simulink model "f_22_stabilator_control - Copy"  (R2025b)
settings: Solver=ode23t  StartTime=0.0  StopTime=10.0  MinStep=1e-8  RelTol=1e-3  AbsTol=1e-6
InitFcn:
  | Running_in_Simulink = 1;
  | 
  | Relation;
values from neighbouring files (symbols this model uses):
  alpha = rad2deg(asin(d/a))    [Relation.m]
  D = 163.1    [EHA_initialization.m]
  deflection = deflection_min:0.01:deflection_max    [Relation.m]
  extension = sqrt(a^2 + r^2 - 2.*a.*r.*cos(deg2rad(alpha-deflection))) - d    [Relation.m]
  F_act = M_pivot ./ lever_arm_actuator    [Relation.m]
  J = 0.205    [EHA_initialization.m]
  K_e = 0.132    [EHA_initialization.m]
  K_vism = 1    [EHA_initialization.m]
  L = 1.95e-5    (= 1.95e-05)    [EHA_initialization.m]
  P_aci = P_acnom    (= 20.7)    [EHA_initialization.m]
  R = 138000/(370^2)    (= 1.00803506209)    [EHA_initialization.m]
  V_gasi = V_gasnom    (= 0.00206)    [EHA_initialization.m]
  velocity = 300    [Relation.m]
undefined symbols (not defined in the file or in its folder): A, B, beta, F_c, F_s, k, K_elp, K_ilj, K_ilp, K_t, K_vis, M, T_c, T_f, V_10, V_20
libraries: slpidlib x3
settings Model: Creator=Arseni  LastModifiedBy=User
settings SolverCC: AutoScaleAbsTol=off  MaxConsecutiveMinStep=10  SolverResetMethod=Robust

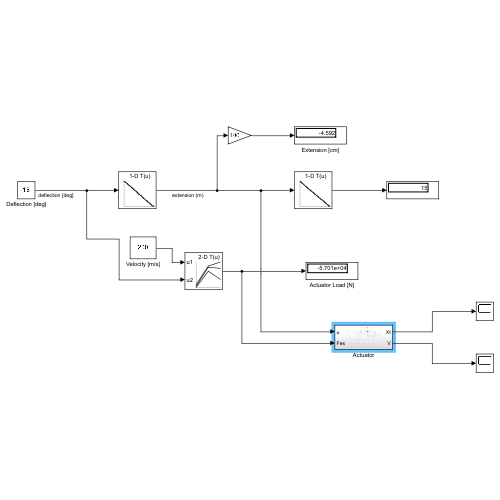
[thumbnail: Simulink's stored preview of the top-level diagram]
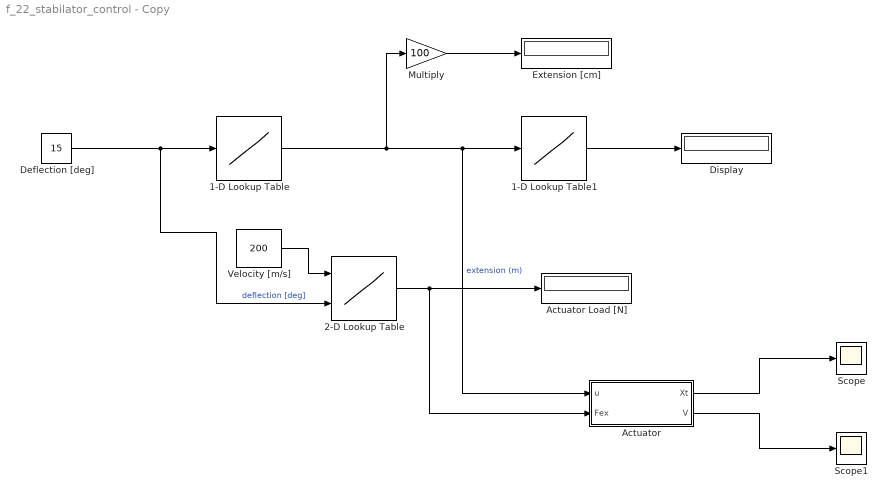
== system f_22_stabilator_control - Copy ==
  1-D Lookup Table : Lookup_n-D  NumberOfTableDimensions=1  BreakpointsForDimension1=deflection  Table=extension  InternalRulePriority=Speed  RndMeth=Simplest
  1-D Lookup Table1 : Lookup_n-D  NumberOfTableDimensions=1  BreakpointsForDimension1=flip(extension)  Table=flip(deflection)  InternalRulePriority=Speed  RndMeth=Simplest
  2-D Lookup Table : Lookup_n-D  BreakpointsForDimension1=velocity  BreakpointsForDimension2=deflection  Table=F_act  InternalRulePriority=Speed  RndMeth=Simplest
      settings: InputPortMap=u0,u1
  Actuator : Subsystem
  Actuator Load [N] : Display
  Deflection [deg] : Constant  Value=15
  Display : Display
  Extension [cm] : Display
  Multiply : Gain  Gain=100
  Scope : Scope
      settings: ActiveDisplayYMinimum=-0.010270198712265704  ActiveDisplayYMaximum=0.016528927509019922
  Scope1 : Scope
      settings: ActiveDisplayYMinimum=-22.309265699882108  ActiveDisplayYMaximum=23.598774285341456
  Velocity [m/s] : Constant  Value=200
  wires:
  Deflection [deg]/1 -> 2-D Lookup Table/2, 1-D Lookup Table/1  "deflection [deg]"
  1-D Lookup Table/1 -> 1-D Lookup Table1/1, Actuator/1(u), Multiply/1  "extension (m)"
  1-D Lookup Table1/1 -> Display/1
  Multiply/1 -> Extension [cm]/1
  2-D Lookup Table/1 -> Actuator Load [N]/1, Actuator/2(Fex)
  Velocity [m/s]/1 -> 2-D Lookup Table/1
  Actuator/1(Xt) -> Scope/1
  Actuator/2(V) -> Scope1/1

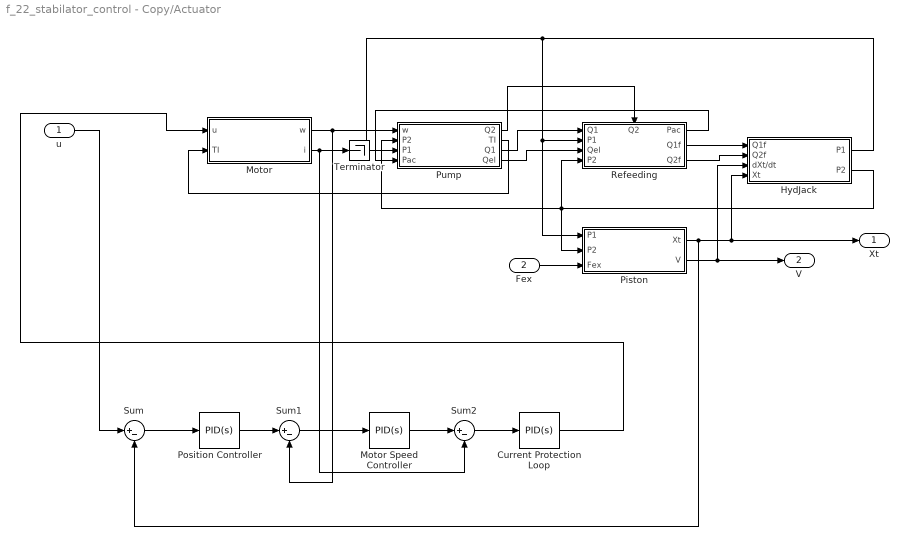
== system f_22_stabilator_control - Copy/Actuator ==
  u : Inport
  Fex : Inport  Port=2
  Current Protection Loop : slpidlib/PID Controller  Controller=PID  Form=Parallel  TimeDomain=Continuous-time  UseExternalTs=off  SampleTime=-1  IntegratorMethod=Forward Euler  FilterMethod=Forward Euler  ControllerParametersSource=internal  P=0.5  I=0  UseKiTs=off  D=0  UseExternalDerivativeSource=off  N=100  UseFilter=on  TunerSelectOption=Transfer Function Based (PID Tuner App)  InitialConditionSource=internal  InitialConditionForIntegrator=0  InitialConditionForFilter=0  DifferentiatorICPrevScaledInput=0  ExternalReset=none  TrackingMode=off  Kt=1  LimitOutput=on  SatLimitsSource=internal  UpperSaturationLimit=270  LowerSaturationLimit=-270  LinearizeAsGain=on  AntiWindupMode=clamping  Kb=1  LimitIntegrator=off  UpperIntegratorSaturationLimit=inf  LowerIntegratorSaturationLimit=-inf  POutMin=[]  POutMax=[]  IOutMin=[]  IOutMax=[]  DOutMin=[]  DOutMax=[]  NOutMin=[]  NOutMax=[]  SumOutMin=[]  SumOutMax=[]  SaturationOutMin=[]  SaturationOutMax=[]  PParamMin=[]  PParamMax=[]  IParamMin=[]  IParamMax=[]  DParamMin=[]  DParamMax=[]  NParamMin=[]  NParamMax=[]  KbParamMin=[]  KbParamMax=[]  KtParamMin=[]  KtParamMax=[]  KbOutMin=[]  KbOutMax=[]  KtOutMin=[]  KtOutMax=[]  IntegratorOutMin=[]  IntegratorOutMax=[]  FilterOutMin=[]  FilterOutMax=[]  SumI1OutMin=[]  SumI1OutMax=[]  SumI2OutMin=[]  SumI2OutMax=[]  SumI3OutMin=[]  SumI3OutMax=[]  SumI4OutMin=[]  SumI4OutMax=[]  SumDOutMin=[]  SumDOutMax=[]  DifferentiatorOutMin=[]  DifferentiatorOutMax=[]  FilterDiffOutCoefMin=[]  FilterDiffOutCoefMax=[]  ReciprocalOutMin=[]  ReciprocalOutMax=[]  SumDenOutMin=[]  SumDenOutMax=[]  SumNumOutMin=[]  SumNumOutMax=[]  DivideOutMin=[]  DivideOutMax=[]  UdiffTsProdOutMin=[]  UdiffTsProdOutMax=[]  NTsProdOutMin=[]  NTsProdOutMax=[]  UintegralTsProdOutMin=[]  UintegralTsProdOutMax=[]  UngainTsProdOutMin=[]  UngainTsProdOutMax=[]  ClampingZeroOutDataTypeStr=Inherit: Inherit via back propagation  ClampingZeroOutMin=[]  ClampingZeroOutMax=[]  FilterDenConstantOutDataTypeStr=Inherit: Inherit via back propagation  FilterDenConstantOutMin=[]  FilterDenConstantOutMax=[]  PCopyOutDataTypeStr=Inherit: Inherit via back propagation  PCopyOutMin=[]  PCopyOutMax=[]  NCopyOutDataTypeStr=Inherit: Inherit via back propagation  NCopyOutMin=[]  NCopyOutMax=[]  IntegratorContinuousStateAttributes=''  IntegratorStateMustResolveToSignalObject=off  IntegratorRTWStateStorageClass=Auto  FilterContinuousStateAttributes=''  FilterStateMustResolveToSignalObject=off  FilterRTWStateStorageClass=Auto  ParallelPVariant=InternalParameters  IdealPVariant=Disabled  IVariant=InternalParameters  DVariant=InternalParameters  IntegratorVariant=Continuous  SatVariant=Enabled  AWVariant=ContClampingParallel  PCopyVariant=Disabled  TRVariant=Disabled  FdbkBlocksVariant=Forward  IdealPFdbkVariant=Disabled  SatFdbkVariant=Disabled  DerivativeFilterVariant=ContFilter  NVariant=InternalParameters  NCopyVariant=Disabled  FilterICVariant=InternalICsFilter  IntegratorICVariant=InternalICs  ExternalResetVariant=Disabled  TRSumVariant=Passthrough  SumFdbkVariant=Disabled  SumVariant=Sum_PID  TsampFilterVariant=InternalTs  TsampNgainVariant=Passthrough  TsampIntegralVariant=Disabled_SignalSpec  ExternalSaturationOutDataTypeStr=Inherit: Same as second input  DerivativeSourceVariant=ErrorSignal  PreIntVariant=InternalPreInt
  HydJack : Subsystem
  Motor : Subsystem
  Motor Speed Controller : slpidlib/PID Controller  Controller=PID  Form=Parallel  TimeDomain=Continuous-time  UseExternalTs=off  SampleTime=-1  IntegratorMethod=Forward Euler  FilterMethod=Forward Euler  ControllerParametersSource=internal  P=5  I=1  UseKiTs=off  D=1  UseExternalDerivativeSource=off  N=100  UseFilter=on  TunerSelectOption=Transfer Function Based (PID Tuner App)  InitialConditionSource=internal  InitialConditionForIntegrator=0  InitialConditionForFilter=0  DifferentiatorICPrevScaledInput=0  ExternalReset=none  TrackingMode=off  Kt=1  LimitOutput=off  SatLimitsSource=internal  UpperSaturationLimit=inf  LowerSaturationLimit=-inf  LinearizeAsGain=on  AntiWindupMode=none  Kb=1  LimitIntegrator=off  UpperIntegratorSaturationLimit=inf  LowerIntegratorSaturationLimit=-inf  POutMin=[]  POutMax=[]  IOutMin=[]  IOutMax=[]  DOutMin=[]  DOutMax=[]  NOutMin=[]  NOutMax=[]  SumOutMin=[]  SumOutMax=[]  SaturationOutMin=[]  SaturationOutMax=[]  PParamMin=[]  PParamMax=[]  IParamMin=[]  IParamMax=[]  DParamMin=[]  DParamMax=[]  NParamMin=[]  NParamMax=[]  KbParamMin=[]  KbParamMax=[]  KtParamMin=[]  KtParamMax=[]  KbOutMin=[]  KbOutMax=[]  KtOutMin=[]  KtOutMax=[]  IntegratorOutMin=[]  IntegratorOutMax=[]  FilterOutMin=[]  FilterOutMax=[]  SumI1OutMin=[]  SumI1OutMax=[]  SumI2OutMin=[]  SumI2OutMax=[]  SumI3OutMin=[]  SumI3OutMax=[]  SumI4OutMin=[]  SumI4OutMax=[]  SumDOutMin=[]  SumDOutMax=[]  DifferentiatorOutMin=[]  DifferentiatorOutMax=[]  FilterDiffOutCoefMin=[]  FilterDiffOutCoefMax=[]  ReciprocalOutMin=[]  ReciprocalOutMax=[]  SumDenOutMin=[]  SumDenOutMax=[]  SumNumOutMin=[]  SumNumOutMax=[]  DivideOutMin=[]  DivideOutMax=[]  UdiffTsProdOutMin=[]  UdiffTsProdOutMax=[]  NTsProdOutMin=[]  NTsProdOutMax=[]  UintegralTsProdOutMin=[]  UintegralTsProdOutMax=[]  UngainTsProdOutMin=[]  UngainTsProdOutMax=[]  ClampingZeroOutDataTypeStr=Inherit: Inherit via back propagation  ClampingZeroOutMin=[]  ClampingZeroOutMax=[]  FilterDenConstantOutDataTypeStr=Inherit: Inherit via back propagation  FilterDenConstantOutMin=[]  FilterDenConstantOutMax=[]  PCopyOutDataTypeStr=Inherit: Inherit via back propagation  PCopyOutMin=[]  PCopyOutMax=[]  NCopyOutDataTypeStr=Inherit: Inherit via back propagation  NCopyOutMin=[]  NCopyOutMax=[]  IntegratorContinuousStateAttributes=''  IntegratorStateMustResolveToSignalObject=off  IntegratorRTWStateStorageClass=Auto  FilterContinuousStateAttributes=''  FilterStateMustResolveToSignalObject=off  FilterRTWStateStorageClass=Auto  ParallelPVariant=InternalParameters  IdealPVariant=Disabled  IVariant=InternalParameters  DVariant=InternalParameters  IntegratorVariant=Continuous  SatVariant=Disabled  AWVariant=Passthrough  PCopyVariant=Disabled  TRVariant=Disabled  FdbkBlocksVariant=Forward  IdealPFdbkVariant=Disabled  SatFdbkVariant=Disabled  DerivativeFilterVariant=ContFilter  NVariant=InternalParameters  NCopyVariant=Disabled  FilterICVariant=InternalICsFilter  IntegratorICVariant=InternalICs  ExternalResetVariant=Disabled  TRSumVariant=Passthrough  SumFdbkVariant=Disabled  SumVariant=Sum_PID  TsampFilterVariant=InternalTs  TsampNgainVariant=Passthrough  TsampIntegralVariant=Disabled_SignalSpec  ExternalSaturationOutDataTypeStr=Inherit: Same as second input  DerivativeSourceVariant=ErrorSignal  PreIntVariant=InternalPreInt
  Piston : Subsystem
  Position Controller : slpidlib/PID Controller  Controller=PID  Form=Parallel  TimeDomain=Continuous-time  UseExternalTs=off  SampleTime=-1  IntegratorMethod=Forward Euler  FilterMethod=Forward Euler  ControllerParametersSource=internal  P=0.5  I=0.1  UseKiTs=off  D=0  UseExternalDerivativeSource=off  N=100  UseFilter=on  TunerSelectOption=Transfer Function Based (PID Tuner App)  InitialConditionSource=internal  InitialConditionForIntegrator=0  InitialConditionForFilter=0  DifferentiatorICPrevScaledInput=0  ExternalReset=none  TrackingMode=off  Kt=1  LimitOutput=off  SatLimitsSource=internal  UpperSaturationLimit=inf  LowerSaturationLimit=-inf  LinearizeAsGain=on  AntiWindupMode=none  Kb=1  LimitIntegrator=off  UpperIntegratorSaturationLimit=inf  LowerIntegratorSaturationLimit=-inf  POutMin=[]  POutMax=[]  IOutMin=[]  IOutMax=[]  DOutMin=[]  DOutMax=[]  NOutMin=[]  NOutMax=[]  SumOutMin=[]  SumOutMax=[]  SaturationOutMin=[]  SaturationOutMax=[]  PParamMin=[]  PParamMax=[]  IParamMin=[]  IParamMax=[]  DParamMin=[]  DParamMax=[]  NParamMin=[]  NParamMax=[]  KbParamMin=[]  KbParamMax=[]  KtParamMin=[]  KtParamMax=[]  KbOutMin=[]  KbOutMax=[]  KtOutMin=[]  KtOutMax=[]  IntegratorOutMin=[]  IntegratorOutMax=[]  FilterOutMin=[]  FilterOutMax=[]  SumI1OutMin=[]  SumI1OutMax=[]  SumI2OutMin=[]  SumI2OutMax=[]  SumI3OutMin=[]  SumI3OutMax=[]  SumI4OutMin=[]  SumI4OutMax=[]  SumDOutMin=[]  SumDOutMax=[]  DifferentiatorOutMin=[]  DifferentiatorOutMax=[]  FilterDiffOutCoefMin=[]  FilterDiffOutCoefMax=[]  ReciprocalOutMin=[]  ReciprocalOutMax=[]  SumDenOutMin=[]  SumDenOutMax=[]  SumNumOutMin=[]  SumNumOutMax=[]  DivideOutMin=[]  DivideOutMax=[]  UdiffTsProdOutMin=[]  UdiffTsProdOutMax=[]  NTsProdOutMin=[]  NTsProdOutMax=[]  UintegralTsProdOutMin=[]  UintegralTsProdOutMax=[]  UngainTsProdOutMin=[]  UngainTsProdOutMax=[]  ClampingZeroOutDataTypeStr=Inherit: Inherit via back propagation  ClampingZeroOutMin=[]  ClampingZeroOutMax=[]  FilterDenConstantOutDataTypeStr=Inherit: Inherit via back propagation  FilterDenConstantOutMin=[]  FilterDenConstantOutMax=[]  PCopyOutDataTypeStr=Inherit: Inherit via back propagation  PCopyOutMin=[]  PCopyOutMax=[]  NCopyOutDataTypeStr=Inherit: Inherit via back propagation  NCopyOutMin=[]  NCopyOutMax=[]  IntegratorContinuousStateAttributes=''  IntegratorStateMustResolveToSignalObject=off  IntegratorRTWStateStorageClass=Auto  FilterContinuousStateAttributes=''  FilterStateMustResolveToSignalObject=off  FilterRTWStateStorageClass=Auto  ParallelPVariant=InternalParameters  IdealPVariant=Disabled  IVariant=InternalParameters  DVariant=InternalParameters  IntegratorVariant=Continuous  SatVariant=Disabled  AWVariant=Passthrough  PCopyVariant=Disabled  TRVariant=Disabled  FdbkBlocksVariant=Forward  IdealPFdbkVariant=Disabled  SatFdbkVariant=Disabled  DerivativeFilterVariant=ContFilter  NVariant=InternalParameters  NCopyVariant=Disabled  FilterICVariant=InternalICsFilter  IntegratorICVariant=InternalICs  ExternalResetVariant=Disabled  TRSumVariant=Passthrough  SumFdbkVariant=Disabled  SumVariant=Sum_PID  TsampFilterVariant=InternalTs  TsampNgainVariant=Passthrough  TsampIntegralVariant=Disabled_SignalSpec  ExternalSaturationOutDataTypeStr=Inherit: Same as second input  DerivativeSourceVariant=ErrorSignal  PreIntVariant=InternalPreInt
  Pump : Subsystem
  Refeeding : Subsystem
      settings: PortSchema="{\"entries\":[{\"content\":{\"sides\":[{\"content\":{\"connectorIds\":[\"In1\",\"In2\",\"In3\",\"In4\"]},\"type\":\"ConnectorPlacement.EquallySpacedRectSide\",\"uuid\":\"b1abc16c-430b-4270-8249-0157d5dcf7da\"},{\"content\":{\"connectorIds\":[\"Out1\",\"Out2\",\"Out3\"],\"side\":\"RIGHT\"},\"type\":\"ConnectorPlacement.EquallySpacedRectSide\",\"uuid\":\"915786c5-2ea2-4759-aadd-eadd86a3997f\"},{\"content\":{\"connectorIds\":[\"In5\"],\"side\":\"TOP\"},\"type\":\"ConnectorPlacement.EquallySpacedRectSide\",\"uuid\":\"af1c57d2-4a41-47dc-aec2-d26e5b158527\"}]},\"type\":\"ConnectorPlacement.EquallySpacedConnector\",\"uuid\":\"dcd4a5ce-5031-43e1-ac08-793124a08eaa\"}],\"packageUris\":[\"http://schema.mathworks.com/mf0/Connector/R2020b\"],\"version\":\"1.0\"}"
  Sum : Sum  Inputs=|+-
  Sum1 : Sum  Inputs=|+-
  Sum2 : Sum  Inputs=|+-
  Terminator : Terminator
  Xt : Outport
  V : Outport  Port=2
  wires:
  Motor/1(w) -> Pump/1(w), Sum1/2
  Motor/2(i) -> Terminator/1, Sum2/2
  Pump/3(Q1) -> Refeeding/1(Q1)
  Pump/1(Q2) -> Refeeding/5(Q2)
  Pump/4(Qel) -> Refeeding/3(Qel)
  Refeeding/1(Pac) -> Pump/4(Pac)
  Pump/2(TI) -> Motor/2(TI)
  Refeeding/2(Q1f) -> HydJack/1(Q1f)
  Refeeding/3(Q2f) -> HydJack/2(Q2f)
  HydJack/1(P1) -> Piston/1(P1), Refeeding/2(P1), Pump/3(P1)
  HydJack/2(P2) -> Refeeding/4(P2), Pump/2(P2), Piston/2(P2)
  Fex/1 -> Piston/3(Fex)
  Piston/1(Xt) -> Xt/1, HydJack/4(Xt), Sum/2
  Piston/2(V) -> V/1, HydJack/3(dXt/dt)
  u/1 -> Sum/1
  Sum/1 -> Position Controller/1
  Position Controller/1 -> Sum1/1
  Sum1/1 -> Motor Speed Controller/1
  Motor Speed Controller/1 -> Sum2/1
  Sum2/1 -> Current Protection Loop/1
  Current Protection Loop/1 -> Motor/1(u)

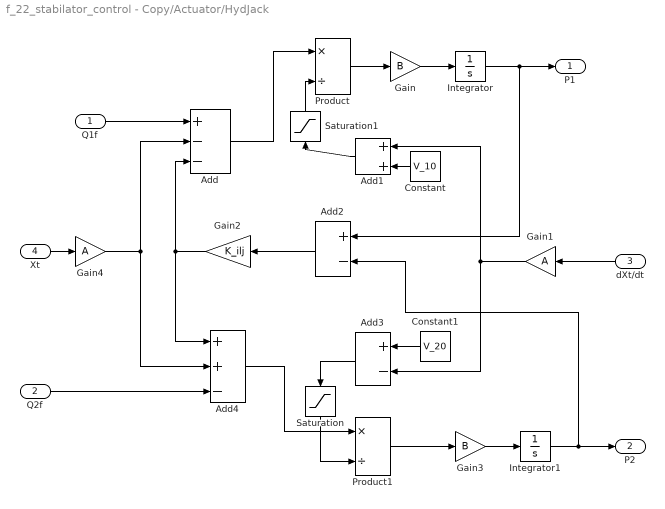
== system f_22_stabilator_control - Copy/Actuator/HydJack ==
  Q1f : Inport
  Q2f : Inport  Port=2
  dXt/dt : Inport  Port=3
  Xt : Inport  Port=4
  Add : Sum  Inputs=+--
  Add1 : Sum
  Add2 : Sum  Inputs=+-
  Add3 : Sum  Inputs=+-
  Add4 : Sum  Inputs=++-
  Constant : Constant  Value=V_10
  Constant1 : Constant  Value=V_20
  Gain : Gain  Gain=B
  Gain1 : Gain  Gain=A
  Gain2 : Gain  Gain=K_ilj
  Gain3 : Gain  Gain=B
  Gain4 : Gain  Gain=A
  Integrator : Integrator  InitialCondition=P_aci
  Integrator1 : Integrator  InitialCondition=P_aci
  Product : Product  Inputs=*/
  Product1 : Product  Inputs=*/
  Saturation : Saturate  UpperLimit=inf  LowerLimit=1e-6
  Saturation1 : Saturate  UpperLimit=inf  LowerLimit=1e-6
  P1 : Outport
  P2 : Outport  Port=2
  wires:
  Q1f/1 -> Add/1
  Add/1 -> Product/1
  Product/1 -> Gain/1
  Gain/1 -> Integrator/1
  Integrator/1 -> Add2/1, P1/1
  dXt/dt/1 -> Gain1/1
  Gain1/1 -> Add1/1, Add3/2
  Constant/1 -> Add1/2
  Add2/1 -> Gain2/1
  Gain2/1 -> Add4/1, Add/3
  Constant1/1 -> Add3/1
  Product1/1 -> Gain3/1
  Gain3/1 -> Integrator1/1
  Integrator1/1 -> Add2/2, P2/1
  Q2f/1 -> Add4/3
  Xt/1 -> Gain4/1
  Gain4/1 -> Add4/2, Add/2
  Add1/1 -> Saturation1/1
  Add4/1 -> Product1/1
  Add3/1 -> Saturation/1
  Saturation/1 -> Product1/2
  Saturation1/1 -> Product/2

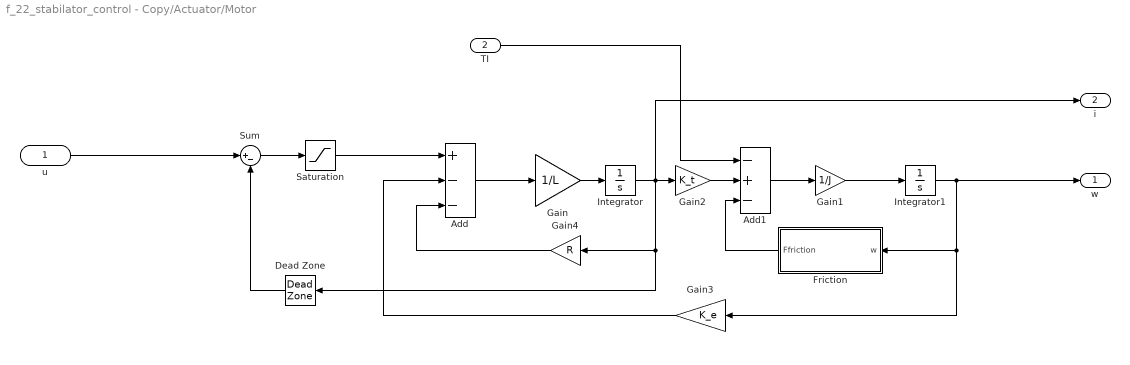
== system f_22_stabilator_control - Copy/Actuator/Motor ==
  u : Inport
  TI : Inport  Port=2
  Add : Sum  Inputs=+--
  Add1 : Sum  Inputs=-+-
  Dead Zone : DeadZone  LowerValue=-3.75  UpperValue=3.75
  Friction : Subsystem
  Gain : Gain  Gain=1/L
  Gain1 : Gain  Gain=1/J
  Gain2 : Gain  Gain=K_t
  Gain3 : Gain  Gain=K_e
  Gain4 : Gain  Gain=R
  Integrator : Integrator
  Integrator1 : Integrator
  Saturation : Saturate  UpperLimit=270  LowerLimit=-270
  Sum : Sum  Inputs=|+-
  w : Outport
  i : Outport  Port=2
  wires:
  Add/1 -> Gain/1
  Gain/1 -> Integrator/1
  Gain1/1 -> Integrator1/1
  Integrator1/1 -> w/1, Gain3/1, Friction/1(w)
  Add1/1 -> Gain1/1
  Integrator/1 -> i/1, Dead Zone/1, Gain4/1, Gain2/1
  Gain2/1 -> Add1/2
  Gain3/1 -> Add/2
  Gain4/1 -> Add/3
  Friction/1(Ffriction) -> Add1/3
  Sum/1 -> Saturation/1
  Saturation/1 -> Add/1
  Dead Zone/1 -> Sum/2
  TI/1 -> Add1/1
  u/1 -> Sum/1

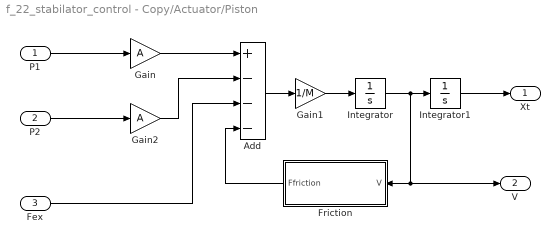
== system f_22_stabilator_control - Copy/Actuator/Piston ==
  P1 : Inport
  P2 : Inport  Port=2
  Fex : Inport  Port=3
  Add : Sum  Inputs=+---
  Friction : Subsystem
  Gain : Gain  Gain=A
  Gain1 : Gain  Gain=1/M
  Gain2 : Gain  Gain=A
  Integrator : Integrator
  Integrator1 : Integrator  LimitOutput=on  UpperSaturationLimit=0.0751  LowerSaturationLimit=-0.0885
  Xt : Outport
  V : Outport  Port=2
  wires:
  P1/1 -> Gain/1
  Gain/1 -> Add/1
  Add/1 -> Gain1/1
  Gain1/1 -> Integrator/1
  Integrator1/1 -> Xt/1
  Integrator/1 -> Integrator1/1, V/1, Friction/1(V)
  P2/1 -> Gain2/1
  Gain2/1 -> Add/2
  Fex/1 -> Add/3
  Friction/1(Ffriction) -> Add/4

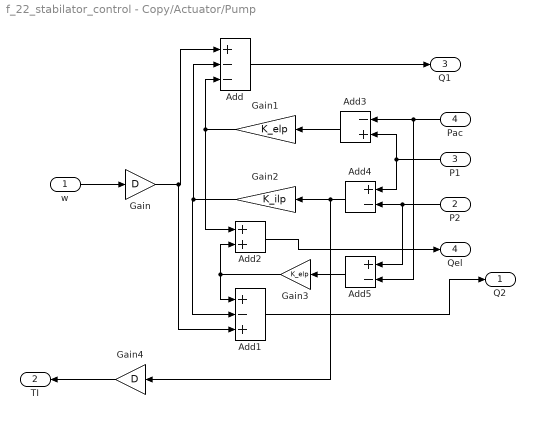
== system f_22_stabilator_control - Copy/Actuator/Pump ==
  w : Inport
  P2 : Inport  Port=2
  P1 : Inport  Port=3
  Pac : Inport  Port=4
  Add : Sum  Inputs=+--
  Add1 : Sum  Inputs=+-+
  Add2 : Sum
  Add3 : Sum  Inputs=-+
  Add4 : Sum  Inputs=+-
  Add5 : Sum  Inputs=+-
  Gain : Gain  Gain=D
  Gain1 : Gain  Gain=K_elp
  Gain2 : Gain  Gain=K_ilp
  Gain3 : Gain  Gain=K_elp
  Gain4 : Gain  Gain=D
  Q2 : Outport
  TI : Outport  Port=2
  Q1 : Outport  Port=3
  Qel : Outport  Port=4
  wires:
  w/1 -> Gain/1
  Gain/1 -> Add1/3, Add/1
  Add/1 -> Q1/1
  Pac/1 -> Add5/2, Add3/1
  Add3/1 -> Gain1/1
  Gain1/1 -> Add2/1, Add/3
  P1/1 -> Add4/1, Add3/2
  P2/1 -> Add5/1, Add4/2
  Add4/1 -> Gain4/1, Gain2/1
  Gain2/1 -> Add/2, Add1/2
  Add5/1 -> Gain3/1
  Gain3/1 -> Add2/2, Add1/1
  Add2/1 -> Qel/1
  Gain4/1 -> TI/1
  Add1/1 -> Q2/1

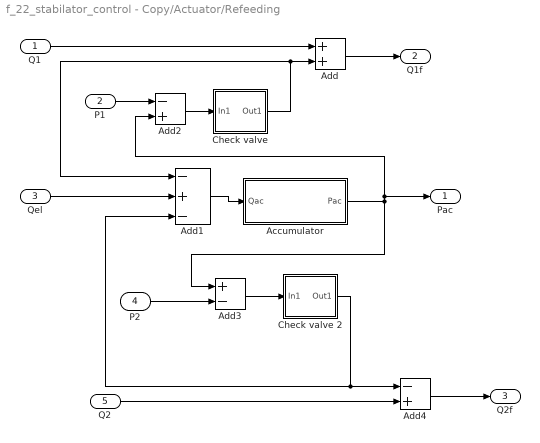
== system f_22_stabilator_control - Copy/Actuator/Refeeding ==
  Q1 : Inport
  P1 : Inport  Port=2
  Qel : Inport  Port=3
  P2 : Inport  Port=4
  Q2 : Inport  Port=5
  Accumulator : Subsystem
  Add : Sum
  Add1 : Sum  Inputs=-+-
  Add2 : Sum  Inputs=-+
  Add3 : Sum  Inputs=+-
  Add4 : Sum  Inputs=-+
  Check valve : Subsystem
  Check valve 2 : Subsystem
  Pac : Outport
  Q1f : Outport  Port=2
  Q2f : Outport  Port=3
  wires:
  Q1/1 -> Add/1
  Add/1 -> Q1f/1
  Qel/1 -> Add1/2
  P1/1 -> Add2/1
  Add1/1 -> Accumulator/1(Qac)
  Accumulator/1(Pac) -> Add2/2, Pac/1, Add3/1
  P2/1 -> Add3/2
  Q2/1 -> Add4/2
  Add2/1 -> Check valve/1(In1)
  Check valve/1(Out1) -> Add/2, Add1/1
  Add3/1 -> Check valve 2/1(In1)
  Check valve 2/1(Out1) -> Add4/1, Add1/3
  Add4/1 -> Q2f/1

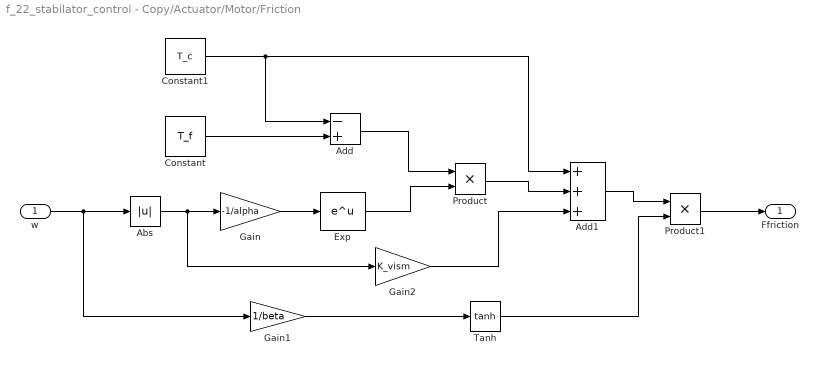
== system f_22_stabilator_control - Copy/Actuator/Motor/Friction ==
  w : Inport
  Abs : Abs  SaturateOnIntegerOverflow=off
  Add : Sum  Inputs=-+
  Add1 : Sum  Inputs=+++
  Constant : Constant  Value=T_f
  Constant1 : Constant  Value=T_c
  Exp : Math
  Gain : Gain  Gain=-1/alpha
  Gain1 : Gain  Gain=1/beta
  Gain2 : Gain  Gain=K_vism
  Product : Product
  Product1 : Product
  Tanh : Trigonometry  Operator=tanh
  Ffriction : Outport
  wires:
  w/1 -> Gain1/1, Abs/1
  Add/1 -> Product/1
  Exp/1 -> Product/2
  Product/1 -> Add1/2
  Add1/1 -> Product1/1
  Product1/1 -> Ffriction/1
  Abs/1 -> Gain2/1, Gain/1
  Gain/1 -> Exp/1
  Gain1/1 -> Tanh/1
  Tanh/1 -> Product1/2
  Gain2/1 -> Add1/3
  Constant/1 -> Add/2
  Constant1/1 -> Add1/1, Add/1

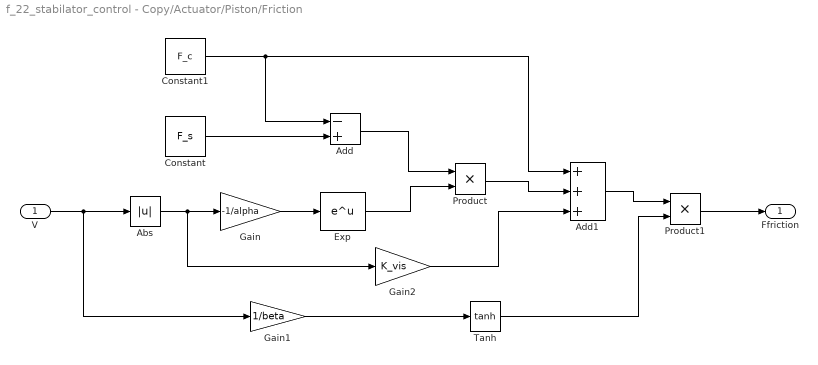
== system f_22_stabilator_control - Copy/Actuator/Piston/Friction ==
  V : Inport
  Abs : Abs  SaturateOnIntegerOverflow=off
  Add : Sum  Inputs=-+
  Add1 : Sum  Inputs=+++
  Constant : Constant  Value=F_s
  Constant1 : Constant  Value=F_c
  Exp : Math
  Gain : Gain  Gain=-1/alpha
  Gain1 : Gain  Gain=1/beta
  Gain2 : Gain  Gain=K_vis
  Product : Product
  Product1 : Product
  Tanh : Trigonometry  Operator=tanh
  Ffriction : Outport
  wires:
  V/1 -> Gain1/1, Abs/1
  Add/1 -> Product/1
  Exp/1 -> Product/2
  Product/1 -> Add1/2
  Add1/1 -> Product1/1
  Product1/1 -> Ffriction/1
  Abs/1 -> Gain2/1, Gain/1
  Gain/1 -> Exp/1
  Gain1/1 -> Tanh/1
  Tanh/1 -> Product1/2
  Gain2/1 -> Add1/3
  Constant/1 -> Add/2
  Constant1/1 -> Add1/1, Add/1

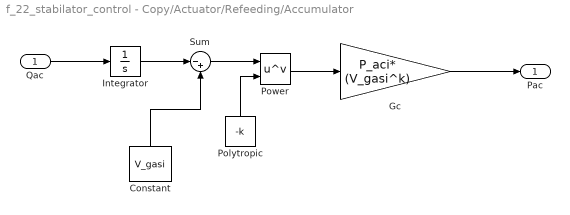
== system f_22_stabilator_control - Copy/Actuator/Refeeding/Accumulator ==
  Qac : Inport
  Constant : Constant  Value=V_gasi
  Gc : Gain  Gain=P_aci* (V_gasi^k)
  Integrator : Integrator
  Polytropic : Constant  Value=-k
  Power : Math  Operator=pow
  Sum : Sum  Inputs=|-+
  Pac : Outport
  wires:
  Qac/1 -> Integrator/1
  Integrator/1 -> Sum/1
  Constant/1 -> Sum/2
  Power/1 -> Gc/1
  Gc/1 -> Pac/1
  Polytropic/1 -> Power/2
  Sum/1 -> Power/1

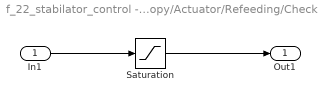
== system f_22_stabilator_control - Copy/Actuator/Refeeding/Check valve ==
  In1 : Inport
  Saturation : Saturate  UpperLimit=inf  LowerLimit=0  ZeroCross=off
      settings: LockScale=on
  Out1 : Outport
  wires:
  In1/1 -> Saturation/1
  Saturation/1 -> Out1/1

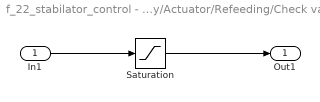
== system f_22_stabilator_control - Copy/Actuator/Refeeding/Check valve 2 ==
  In1 : Inport
  Saturation : Saturate  UpperLimit=inf  LowerLimit=0  ZeroCross=off
      settings: LockScale=on
  Out1 : Outport
  wires:
  In1/1 -> Saturation/1
  Saturation/1 -> Out1/1
